simulink model "genpath_user_iface_ac"  (R2022a)
settings: Solver=FixedStepDiscrete  StartTime=0.0  StopTime=inf  RelTol=1e-3  EnableMultiTasking=on
undefined symbols (not defined in the file or in its folder): HW_BLDC_LQ, HW_BLDC_RS, HW_LOG_VEC_SIZE
libraries: mcbcontrolslib x5, instrumentseriallib x3, svdutilitieslib x1
settings Model: SimulationMode=accelerator  Creator=61301765  LastModifiedBy=61301765
settings OptimizationCC: DefaultParameterBehavior=Inlined  DefaultUnderspecifiedDataType=single  EnhancedBackFolding=on  PassReuseOutputArgsAs=Individual arguments  ZeroExternalMemoryAtStartup=off  MaxStackSize=64  OptimizeBlockOrder=speed  DifferentSizesBufferReuse=on  OptimizationCustomize=off  EfficientTunableParamExpr=on
settings DebuggingCC: ParameterTunabilityLossMsg=error  UnconnectedInputMsg=warning  UnconnectedOutputMsg=warning  UnconnectedLineMsg=warning
settings HardwareCC: ProdBitPerChar=16  ProdBitPerInt=16  ProdBitPerPointer=32  ProdBitPerSizeT=32  ProdBitPerPtrDiffT=32  ProdLargestAtomicInteger=Integer  ProdLargestAtomicFloat=None  ProdWordSize=16  ProdLongLongMode=on  ProdHWDeviceType=Texas Instruments->C2000
settings SFSimCC: MATLABDynamicMemAlloc=off
settings RTWCC: SystemTargetFile=ert.tlc  TemplateMakefile=ert_default_tmf  Toolchain=Texas Instruments Code Composer Studio (C2000)  DLArmComputeVersion=19.05
settings CodeAppCC: ForceParamTrailComments=on  IgnoreCustomStorageClasses=off  OperatorAnnotations=on  SimulinkDataObjDesc=on  SFDataObjDesc=on  InsertBlockDesc=on
settings ERTTargetCC: ExtModeStaticAllocSize=5000  ERTCustomFileTemplate=example_file_process.tlc

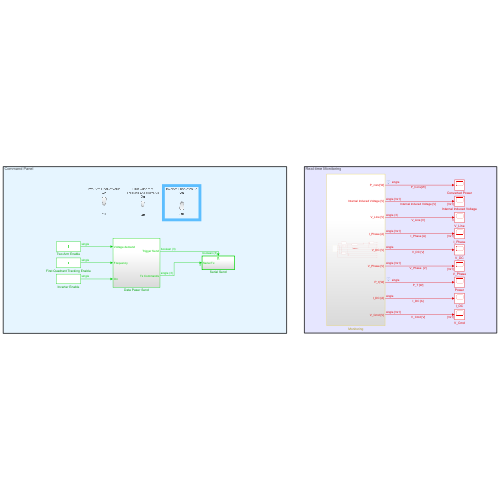
[thumbnail: Simulink's stored preview of the top-level diagram]
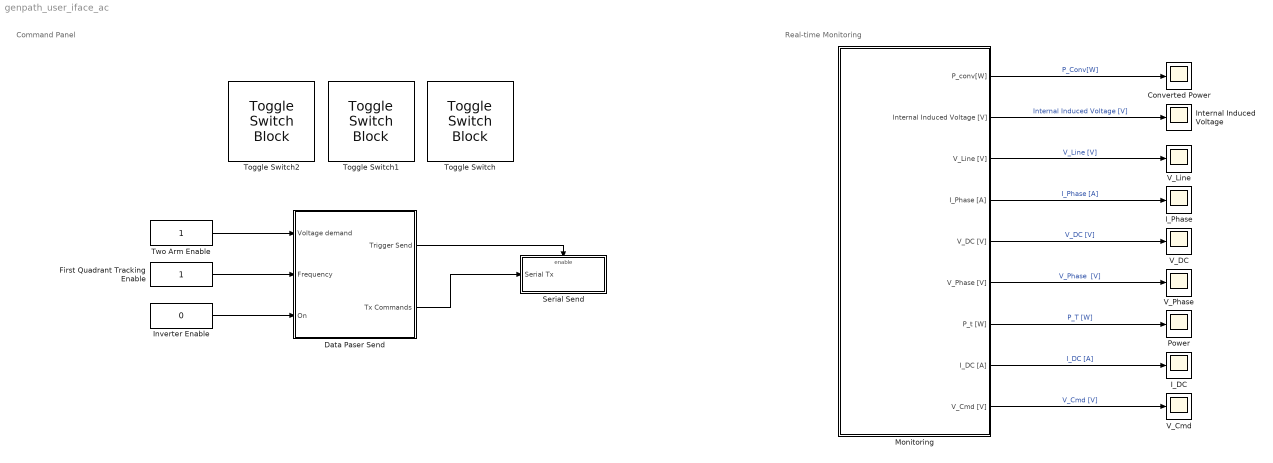
== system genpath_user_iface_ac ==
  note: Real-time Monitoring
  note: Command Panel
  Converted Power : Scope
  Data Paser Send : Subsystem
  First Quadrant Tracking Enable : Constant  VectorParams1D=off  OutDataTypeStr=single  SampleTime=-1
  I_DC : Scope
  I_Phase : Scope
  Internal Induced Voltage : Scope
  Inverter Enable : Constant  Value=0  VectorParams1D=off  OutDataTypeStr=single  SampleTime=-1
  Monitoring : Subsystem
  Power : Scope
  Serial Send : Subsystem  TreatAsAtomicUnit=on
  Toggle Switch : ToggleSwitchBlock
      settings: Values={{'Off', 'On'}, [0 1]}
  Toggle Switch1 : ToggleSwitchBlock
      settings: Values={{'Off', 'On'}, [0 1]}
  Toggle Switch2 : ToggleSwitchBlock
      settings: Values={{'Off', 'On'}, [0 1]}
  Two Arm Enable : Constant  VectorParams1D=off  OutDataTypeStr=single  SampleTime=0.05
  V_Cmd : Scope
  V_DC : Scope
  V_Line : Scope
  V_Phase : Scope
  wires:
  Data Paser Send/2(Tx Commands) -> Serial Send/1(Serial Tx)
  Data Paser Send/1(Trigger Send) -> Serial Send/Enable
  Inverter Enable/1 -> Data Paser Send/3(On)
  Two Arm Enable/1 -> Data Paser Send/1(Voltage demand)
  First Quadrant Tracking Enable/1 -> Data Paser Send/2(Frequency)
  Monitoring/1(P_conv[W]) -> Converted Power/1  "P_Conv[W]"
  Monitoring/3(V_Line [V]) -> V_Line/1  "V_Line [V]"
  Monitoring/4(I_Phase [A]) -> I_Phase/1  "I_Phase [A]"
  Monitoring/5(V_DC [V]) -> V_DC/1  "V_DC [V]"
  Monitoring/6(V_Phase [V]) -> V_Phase/1  "V_Phase  [V]"
  Monitoring/7(P_t [W]) -> Power/1  "P_T [W]"
  Monitoring/8(I_DC [A]) -> I_DC/1  "I_DC [A]"
  Monitoring/2(Internal Induced Voltage [V]) -> Internal Induced Voltage/1  "Internal Induced Voltage [V]"
  Monitoring/9(V_Cmd [V]) -> V_Cmd/1  "V_Cmd [V]"

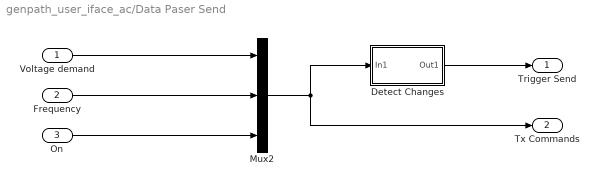
== system genpath_user_iface_ac/Data Paser Send ==
  Voltage demand : Inport
  Frequency : Inport  Port=2
  On : Inport  Port=3
  Detect Changes : Subsystem
  Mux2 : Mux  Inputs=3
  Trigger Send : Outport  VectorParamsAs1DForOutWhenUnconnected=off
  Tx Commands : Outport  Port=2  VectorParamsAs1DForOutWhenUnconnected=off
  wires:
  Mux2/1 -> Tx Commands/1, Detect Changes/1(In1)
  Detect Changes/1(Out1) -> Trigger Send/1
  On/1 -> Mux2/3
  Voltage demand/1 -> Mux2/1
  Frequency/1 -> Mux2/2

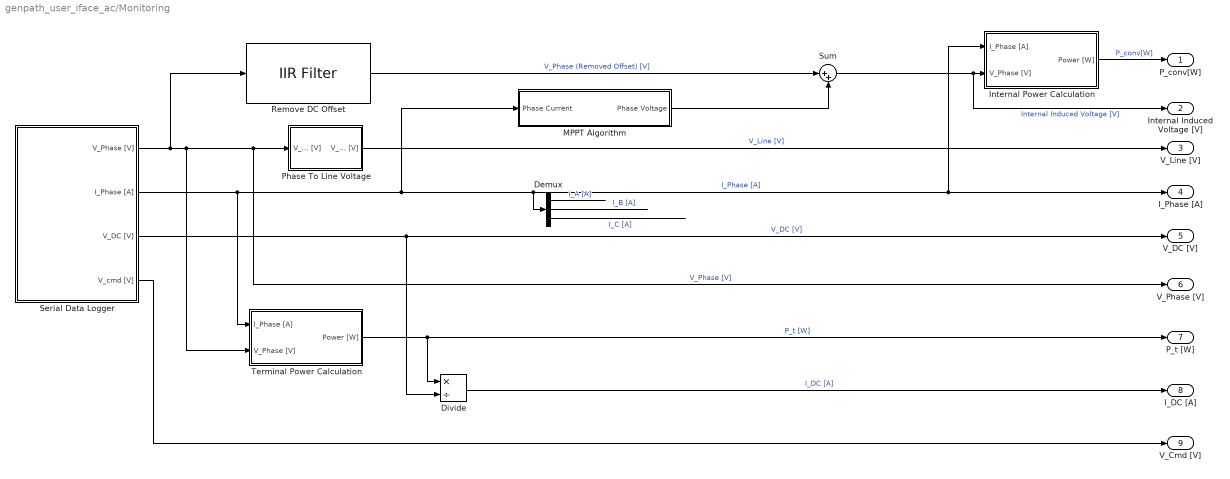
== system genpath_user_iface_ac/Monitoring ==
  Demux : Demux  Outputs=3
  Divide : Product  Inputs=*/
  Internal Power Calculation : Subsystem
  MPPT Algorithm : Subsystem
  Phase To Line Voltage : Subsystem
  Remove DC Offset : mcbcontrolslib/IIR Filter  VariantControl=Low Pass Filter  VariantSelect=High-pass  Filter_constant=0.001  advancedSettings=on  Ts=100e-6  cutOff_freq=1.5931
      settings: SourceProductBaseCode=MT
  Serial Data Logger : Subsystem
  Sum : Sum  Inputs=|++
  Terminal Power Calculation : Subsystem
  P_conv[W] : Outport
  Internal Induced Voltage [V] : Outport  Port=2
  V_Line [V] : Outport  Port=3
  I_Phase [A] : Outport  Port=4
  V_DC [V] : Outport  Port=5
  V_Phase [V] : Outport  Port=6
  P_t [W] : Outport  Port=7
  I_DC [A] : Outport  Port=8
  V_Cmd [V] : Outport  Port=9
  wires:
  Terminal Power Calculation/1(Power [W]) -> P_t [W]/1, Divide/1  "P_t [W]"
  Serial Data Logger/2(I_Phase [A]) -> Terminal Power Calculation/1(I_Phase [A]), MPPT Algorithm/1(Phase Current), Demux/1, I_Phase [A]/1, Internal Power Calculation/1(I_Phase [A])  "I_Phase [A]"
  Serial Data Logger/1(V_Phase [V]) -> Terminal Power Calculation/2(V_Phase [V]), V_Phase [V]/1, Phase To Line Voltage/1(V_Phase [V]), Remove DC Offset/1  "V_Phase [V]"
  Phase To Line Voltage/1(V_Line [V]) -> V_Line [V]/1  "V_Line [V]"
  Serial Data Logger/3(V_DC [V]) -> Divide/2, V_DC [V]/1  "V_DC [V]"
  MPPT Algorithm/1(Phase Voltage) -> Sum/2
  Remove DC Offset/1 -> Sum/1  "V_Phase (Removed Offset) [V]"
  Sum/1 -> Internal Induced Voltage [V]/1, Internal Power Calculation/2(V_Phase [V])  "Internal Induced Voltage [V]"
  Divide/1 -> I_DC [A]/1  "I_DC [A]"
  Internal Power Calculation/1(Power [W]) -> P_conv[W]/1  "P_conv[W]"
  Serial Data Logger/4(V_cmd [V]) -> V_Cmd [V]/1
  Demux/1 -> ?  "I_A [A]"
  Demux/2 -> ?  "I_B [A]"
  Demux/3 -> ?  "I_C [A]"

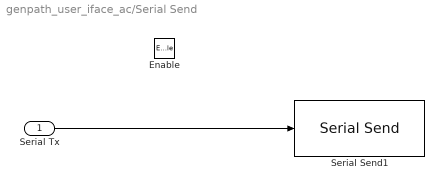
== system genpath_user_iface_ac/Serial Send ==
  Serial Tx : Inport
  Enable : EnablePort
  Serial Send1 : instrumentseriallib/Serial Send  PortSel=COM8  Port=COM8  ComPort=COM8  Header=[ 83 ]  Terminator=Custom terminator  CustomTerminator=[ 69 ]  EnableBlockingMode=on  SimulateUsing=Interpreted execution  BlockInModel=on  aMode=1
      settings: SourceProductBaseCode=OT,IC,MT
  wires:
  Serial Tx/1 -> Serial Send1/1

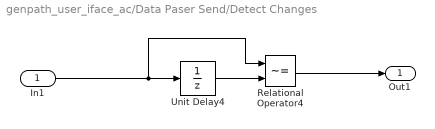
== system genpath_user_iface_ac/Data Paser Send/Detect Changes ==
  In1 : Inport
  Relational Operator4 : RelationalOperator  Operator=~=  OutDataTypeStr=boolean  InputSameDT=off
  Unit Delay4 : UnitDelay  SampleTime=-1  HasFrameUpgradeWarning=on
  Out1 : Outport  VectorParamsAs1DForOutWhenUnconnected=off
  wires:
  Unit Delay4/1 -> Relational Operator4/2
  In1/1 -> Relational Operator4/1, Unit Delay4/1
  Relational Operator4/1 -> Out1/1

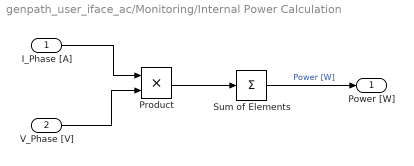
== system genpath_user_iface_ac/Monitoring/Internal Power Calculation ==
  I_Phase [A] : Inport
  V_Phase [V] : Inport  Port=2
  Product : Product
  Sum of Elements : Sum  Inputs=+
  Power [W] : Outport
  wires:
  Sum of Elements/1 -> Power [W]/1  "Power [W]"
  Product/1 -> Sum of Elements/1
  V_Phase [V]/1 -> Product/2
  I_Phase [A]/1 -> Product/1

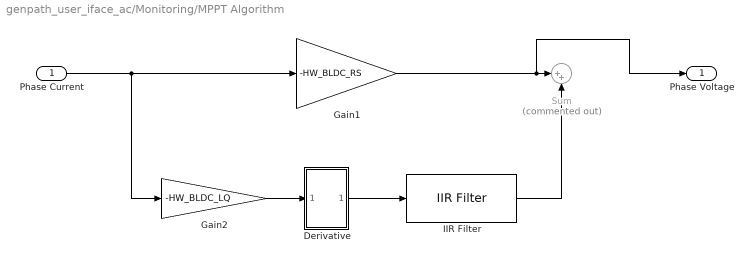
== system genpath_user_iface_ac/Monitoring/MPPT Algorithm ==
  Phase Current : Inport
  Derivative : Subsystem
  Gain1 : Gain  Gain=-HW_BLDC_RS
  Gain2 : Gain  Gain=-HW_BLDC_LQ
  IIR Filter : mcbcontrolslib/IIR Filter  VariantControl=Low Pass Filter  VariantSelect=Low-pass  Filter_constant=0.2  advancedSettings=on  Ts=100e-6  cutOff_freq=397.8874
      settings: SourceProductBaseCode=MT
  Sum : Sum  Commented=on  Inputs=|++
  Phase Voltage : Outport
  wires:
  Phase Current/1 -> Gain2/1, Gain1/1
  Gain1/1 -> Phase Voltage/1, Sum/1
  IIR Filter/1 -> Sum/2
  Gain2/1 -> Derivative/1(In3)
  Derivative/1(Out1) -> IIR Filter/1

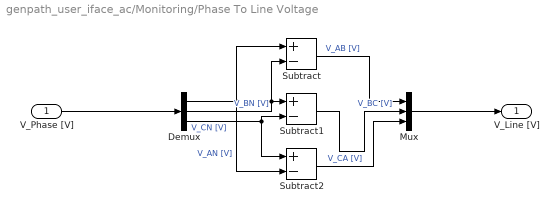
== system genpath_user_iface_ac/Monitoring/Phase To Line Voltage ==
  V_Phase [V] : Inport
  Demux : Demux  Outputs=3
  Mux : Mux  Inputs=3
  Subtract : Sum  Inputs=+-
  Subtract1 : Sum  Inputs=+-
  Subtract2 : Sum  Inputs=+-
  V_Line [V] : Outport
  wires:
  Demux/1 -> Subtract2/2, Subtract/1  "V_AN [V]"
  V_Phase [V]/1 -> Demux/1
  Subtract/1 -> Mux/1  "V_AB [V]"
  Mux/1 -> V_Line [V]/1
  Demux/2 -> Subtract/2, Subtract1/1  "V_BN [V]"
  Subtract1/1 -> Mux/2  "V_BC [V]"
  Subtract2/1 -> Mux/3  "V_CA [V]"
  Demux/3 -> Subtract1/2, Subtract2/1  "V_CN [V]"

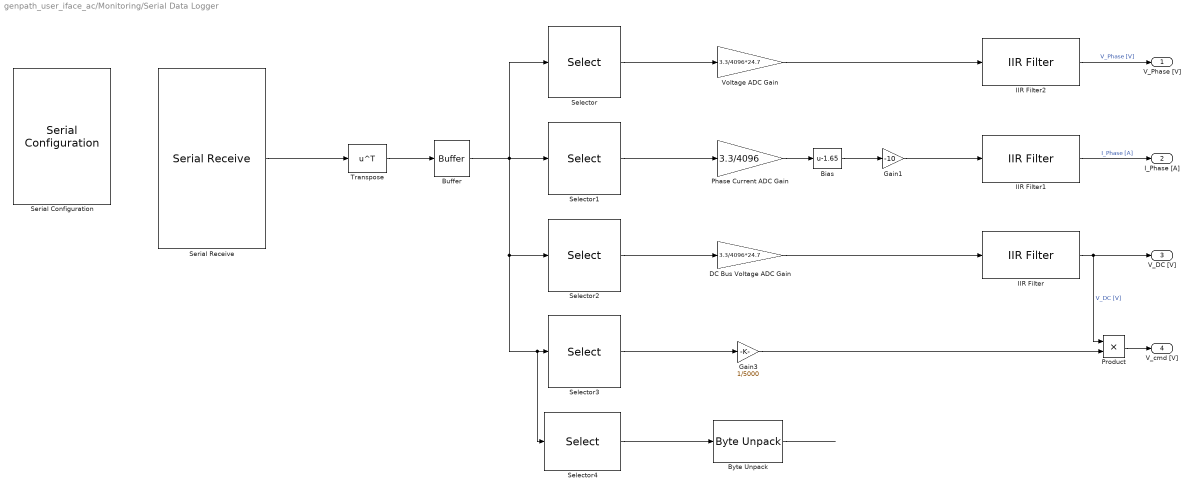
== system genpath_user_iface_ac/Monitoring/Serial Data Logger ==
  Bias : Bias  Bias=-1.65  SaturateOnIntegerOverflow=off
  Buffer : Buffer  N=HW_LOG_VEC_SIZE  OutputFrames=off
  Byte Unpack : svdutilitieslib/Byte Unpack  dimensions={[3]}  datatypes={'single'}  byteAlign=2  blockPlatform=arduinoert
      settings: SourceProductBaseCode=ANDROID,ARDUINO,ML_ARDUINO,ECCORTEXA,ECCORTEXR,SC_BEAGLEBONE_BLUE,EC_FREEDOM_BOARD,EC_FRDM_K64F,INTEL_BLOCKSET,MICROBIT,NUCLEO,NVIDIA,PX4AUTOPILOTS,RASPPIIO,STMICRODIS,TIC2000,XILINX_BLOCKSET
  DC Bus Voltage ADC Gain : Gain  Gain=3.3/4096*24.7  OutDataTypeStr=single
  Gain1 : Gain  Gain=-10
  Gain3 : Gain  Gain=1/5000
  IIR Filter : mcbcontrolslib/IIR Filter  VariantControl=Low Pass Filter  VariantSelect=Low-pass  Filter_constant=0.02  advancedSettings=on  Ts=50e-6  cutOff_freq=64.9612
      settings: SourceProductBaseCode=MT
  IIR Filter1 : mcbcontrolslib/IIR Filter  VariantControl=Low Pass Filter  VariantSelect=Low-pass  Filter_constant=0.02  advancedSettings=on  Ts=50e-6  cutOff_freq=64.9612
      settings: SourceProductBaseCode=MT
  IIR Filter2 : mcbcontrolslib/IIR Filter  VariantControl=Low Pass Filter  VariantSelect=Low-pass  Filter_constant=0.5  advancedSettings=on  Ts=50e-6  cutOff_freq=3183.0989
      settings: SourceProductBaseCode=MT
  Phase Current ADC Gain : Gain  Gain=3.3/4096  OutDataTypeStr=single
  Product : Product
  Selector : Selector  InputPortWidth=HW_LOG_VEC_SIZE  IndexOptions=Index vector (dialog)  Indices=[1 2 3]  OutputSizes=1
  Selector1 : Selector  InputPortWidth=HW_LOG_VEC_SIZE  IndexOptions=Index vector (dialog)  Indices=[4 5 6]  OutputSizes=1
  Selector2 : Selector  InputPortWidth=HW_LOG_VEC_SIZE  IndexOptions=Index vector (dialog)  Indices=7  OutputSizes=1
  Selector3 : Selector  InputPortWidth=HW_LOG_VEC_SIZE  IndexOptions=Index vector (dialog)  Indices=[8 9 10]  OutputSizes=1
  Selector4 : Selector  InputPortWidth=HW_LOG_VEC_SIZE  IndexOptions=Index vector (dialog)  Indices=(11:16)  OutputSizes=1
  Serial Configuration : instrumentseriallib/Serial Configuration  Priority=-200000  PortSel=COM8  Port=COM8  ComPort=COM8  BaudRate=6250000  DataBits=8  Parity=none  StopBits=1  ByteOrder=little-endian  FlowControl=none  Timeout=1  SimulateUsing=Interpreted execution  BlockInModel=on  aMode=1
      settings: SourceProductBaseCode=OT,IC,MT
  Serial Receive : instrumentseriallib/Serial Receive  PortSel=COM8  Port=COM8  ComPort=COM8  DataType=uint16  SaveDataType=uint8  ToggleHeader=on  Header=[238 238]  ToggleTerminator=on  Terminator=Custom terminator  CustomTerminator=[255 255]  InputFormat=Column major  ToggleDataSize=on  DataSize="[1  1000*HW_LOG_VEC_SIZE]"  EnableBlockingMode=on  ActionDataUnavailable=Output last received value  ActionWhenDataUnavailable=Output last received value  CustomValue=0  SampleTime=0.1  SimulateUsing=Interpreted execution  BlockInModel=on  aMode=1
      settings: SourceProductBaseCode=OT,IC,MT
  Transpose : Math  Operator=transpose  SignedPower=on
  Voltage ADC Gain : Gain  Gain=3.3/4096*24.7  OutDataTypeStr=single
  V_Phase [V] : Outport
  I_Phase [A] : Outport  Port=2
  V_DC [V] : Outport  Port=3
  V_cmd [V] : Outport  Port=4
  wires:
  Serial Receive/1 -> Transpose/1
  Buffer/1 -> Selector2/1, Selector4/1, Selector3/1, Selector1/1, Selector/1
  Gain1/1 -> IIR Filter1/1
  Voltage ADC Gain/1 -> IIR Filter2/1
  Selector/1 -> Voltage ADC Gain/1
  IIR Filter/1 -> Product/1, V_DC [V]/1  "V_DC [V]"
  Selector3/1 -> Gain3/1
  Bias/1 -> Gain1/1
  IIR Filter1/1 -> I_Phase [A]/1  "I_Phase [A]"
  Phase Current ADC Gain/1 -> Bias/1
  Transpose/1 -> Buffer/1
  IIR Filter2/1 -> V_Phase [V]/1  "V_Phase [V]"
  Gain3/1 -> Product/2
  Product/1 -> V_cmd [V]/1
  Selector1/1 -> Phase Current ADC Gain/1
  Selector2/1 -> DC Bus Voltage ADC Gain/1
  DC Bus Voltage ADC Gain/1 -> IIR Filter/1
  Selector4/1 -> Byte Unpack/1
  Byte Unpack/1 -> ?

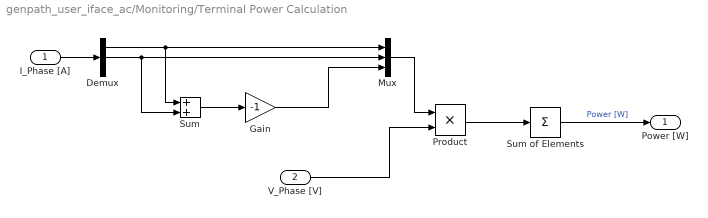
== system genpath_user_iface_ac/Monitoring/Terminal Power Calculation ==
  I_Phase [A] : Inport
  V_Phase [V] : Inport  Port=2
  Demux : Demux  Outputs=3
  Gain : Gain  Gain=-1
  Mux : Mux  Inputs=3
  Product : Product
  Sum : Sum  Inputs=|++
  Sum of Elements : Sum  Inputs=+
  Power [W] : Outport
  wires:
  Sum of Elements/1 -> Power [W]/1  "Power [W]"
  Product/1 -> Sum of Elements/1
  V_Phase [V]/1 -> Product/2
  I_Phase [A]/1 -> Demux/1
  Demux/1 -> Sum/1, Mux/1
  Demux/2 -> Mux/2, Sum/2
  Mux/1 -> Product/1
  Sum/1 -> Gain/1
  Gain/1 -> Mux/3

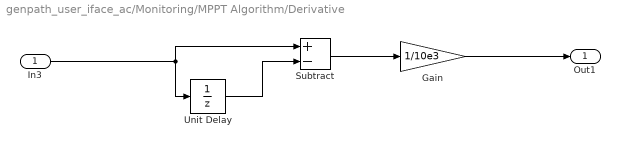
== system genpath_user_iface_ac/Monitoring/MPPT Algorithm/Derivative ==
  In3 : Inport
  Gain : Gain  Gain=1/10e3
  Subtract : Sum  Inputs=+-
  Unit Delay : UnitDelay  SampleTime=-1  HasFrameUpgradeWarning=on
  Out1 : Outport
  wires:
  In3/1 -> Unit Delay/1, Subtract/1
  Unit Delay/1 -> Subtract/2
  Subtract/1 -> Gain/1
  Gain/1 -> Out1/1
